simulink library "HDL_ieee_8021513"  (R2024a)
settings: Solver=FixedStepDiscrete  StartTime=0.0  StopTime=10.0  RelTol=1e-3
undefined symbols (not defined in the file or in its folder): Add, axiWidth, channelCyclicPrefixLen, channelDataCarriers, channelEstReference, channelLUT, channelOFDMSamples, channelScramblerInit, decimatorDelay, decimatorFilter, fPHY, frequencyOffsetTimeWindow, fs, headerBitsPerFec, headerBitsPerOFDMSymbol, headerBitsPerSubcarrier, headerCyclicPrefixLen, headerDataCarriers, headerOFDMSamples, headerScramblerInit, interpolatorDelay, interpolatorFilter, leftGuard, N, ncoCarrierFrequency, ncoWordLength, numDataCarriers, oversamplingFactor, payloadBitsPerFec, payloadScramblerInit, payloadWordsPerBlock0, peakDetectorThreshold, peakDetectorWindow, preambleCyclicPrefixLen, preambleDataCarriers, preambleLUT, preambleOFDMSamples, preambleScramblerInit, QAM, rightGuard, Shift
libraries: hdlsllib x198, $bdroot x80, whdlutilities x28, whdledac x10, whdlmod x7, simulink x4, dsphdlfiltering2 x2, dsphdlsigops2 x2, commhdlcrc x2, dspsigops x2, dspstat3 x2, commdigbbndam3 x2
(part 2 of 5)

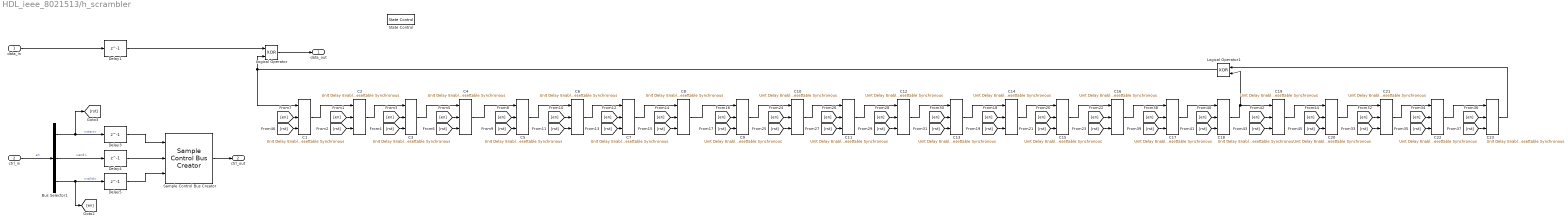
== system HDL_ieee_8021513/h_scrambler ==
  data_in : Inport
  ctrl_in : Inport  Port=2
  Bus Selector1 : BusSelector  OutputSignals=start,end,valid
  C{1,3,5,7,9,11,13,15,17,19,21,23} (12 alike) : hdlsllib/Discrete/Unit Delay Enabled Resettable Synchronous  InitialCondition=0  SampleTime=-1
  C{2,4,6,8,10,12,14,16,18,20,22} (11 alike) : hdlsllib/Discrete/Unit Delay Enabled Resettable Synchronous  InitialCondition=1  SampleTime=-1
  Delay{1,3..5} (4 alike) : Delay  DelayLength=1  InitialCondition=0  UseCircularBuffer=on
  Logical Operator : Logic  Operator=XOR  IconShape=distinctive  AllPortsSameDT=off  OutDataTypeStr=boolean
  Logical Operator1 : Logic  Operator=XOR  IconShape=distinctive  AllPortsSameDT=off  OutDataTypeStr=boolean
  Sample Control Bus Creator : whdlutilities/Sample Control Bus Creator
  State Control : StateControl  StateControl=Synchronous
  data_out : Outport
  ctrl_out : Outport  Port=2  VectorParamsAs1DForOutWhenUnconnected=off
  wires:
  Sample Control Bus Creator/1 -> ctrl_out/1
  Delay5/1 -> Sample Control Bus Creator/3
  Delay4/1 -> Sample Control Bus Creator/2
  Delay3/1 -> Sample Control Bus Creator/1
  Bus Selector1/3 -> Delay5/1, [en]  "<valid>"
  Bus Selector1/2 -> Delay4/1  "<end>"
  Bus Selector1/1 -> Delay3/1, [rst]  "<start>"
  C23/1 -> Logical Operator1/1
  [rst] -> C22/3
  C19/1 -> C20/1
  [en] -> C20/2
  [en] -> C21/2
  C21/1 -> C22/1
  [rst] -> C18/3
  [en] -> C17/2
  [rst] -> C19/3
  [rst] -> C21/3
  C17/1 -> C18/1
  C22/1 -> C23/1
  [en] -> C19/2
  [en] -> C18/2
  [en] -> C23/2
  [rst] -> C20/3
  [en] -> C22/2
  C16/1 -> C17/1
  [rst] -> C23/3
  [rst] -> C17/3
  C8/1 -> C9/1
  [rst] -> C15/3
  [en] -> C15/2
  [en] -> C14/2
  [rst] -> C16/3
  [en] -> C12/2
  [rst] -> C14/3
  C13/1 -> C14/1
  C11/1 -> C12/1
  [rst] -> C9/3
  [en] -> C10/2
  [en] -> C9/2
  C14/1 -> C15/1
  [en] -> C11/2
  [rst] -> C13/3
  C10/1 -> C11/1
  [rst] -> C10/3
  C12/1 -> C13/1
  [en] -> C13/2
  [rst] -> C11/3
  [en] -> C16/2
  [rst] -> C12/3
  C9/1 -> C10/1
  C15/1 -> C16/1
  [rst] -> C5/3
  [en] -> C6/2
  C6/1 -> C7/1
  [en] -> C8/2
  [rst] -> C6/3
  C5/1 -> C6/1
  [rst] -> C7/3
  C7/1 -> C8/1
  [rst] -> C8/3
  [en] -> C7/2
  [en] -> C5/2
  Delay1/1 -> Logical Operator/1
  data_in/1 -> Delay1/1
  ctrl_in/1 -> Bus Selector1/1  "en"
  Logical Operator/1 -> data_out/1
  [rst] -> C3/3
  [en] -> C3/2
  Logical Operator1/1 -> Logical Operator/2, C1/1
  [rst] -> C2/3
  C1/1 -> C2/1
  C3/1 -> C4/1
  [en] -> C1/2
  [rst] -> C1/3
  C4/1 -> C5/1
  [en] -> C4/2
  C2/1 -> C3/1
  [rst] -> C4/3
  [en] -> C2/2
  C20/1 -> C21/1
  C18/1 -> Logical Operator1/2, C19/1

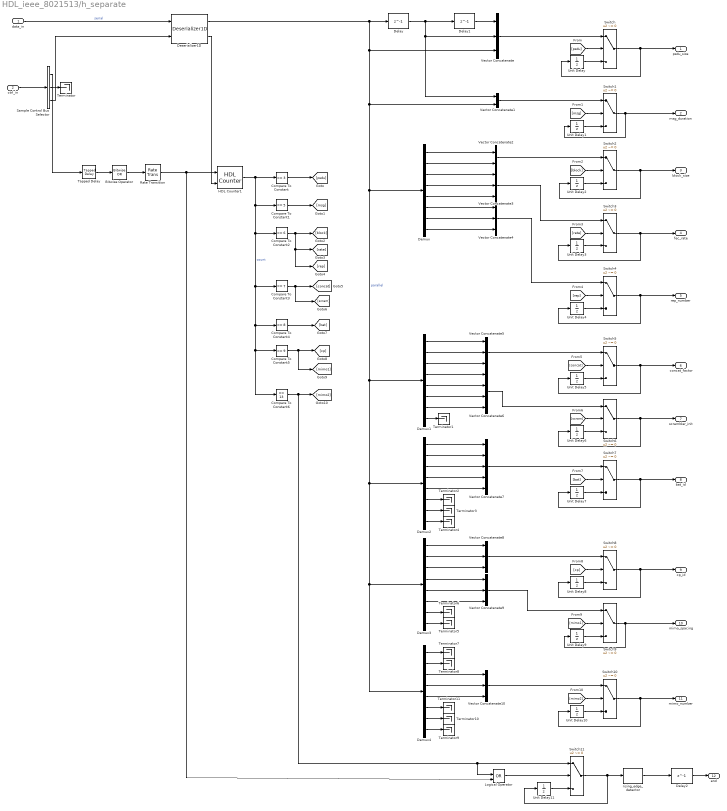
== system HDL_ieee_8021513/h_separate ==
  data_in : Inport
  ctrl_in : Inport  Port=2
  Bitwise Operator : simulink/Logic and Bit Operations/Bitwise Operator  logicop=OR  UseBitMask=off  BitMask=bin2dec('11011001')  BitMaskRealWorld=Stored Integer
      settings: LibrarySourceBlock=|
      | hdlsllib/Logic and Bit
      | Operations/Bitwise
      | Operator
  Compare To Constant : hdlsllib/Logic and Bit Operations/Compare To Constant  relop===  const=3  OutDataTypeStr=boolean
  Compare To Constant1 : hdlsllib/Logic and Bit Operations/Compare To Constant  relop===  const=5  OutDataTypeStr=boolean
  Compare To Constant2 : hdlsllib/Logic and Bit Operations/Compare To Constant  relop===  const=6  OutDataTypeStr=boolean
  Compare To Constant3 : hdlsllib/Logic and Bit Operations/Compare To Constant  relop===  const=7  OutDataTypeStr=boolean
  Compare To Constant4 : hdlsllib/Logic and Bit Operations/Compare To Constant  relop===  const=8  OutDataTypeStr=boolean
  Compare To Constant5 : hdlsllib/Logic and Bit Operations/Compare To Constant  relop===  const=9  OutDataTypeStr=boolean
  Compare To Constant6 : hdlsllib/Logic and Bit Operations/Compare To Constant  relop===  const=13  OutDataTypeStr=boolean
  Delay : Delay  DelayLength=1  InitialCondition=0  UseCircularBuffer=on
  Delay1 : Delay  DelayLength=1  InitialCondition=0  UseCircularBuffer=on
  Delay2 : Delay  DelayLength=1  InitialCondition=0  UseCircularBuffer=on
  Demux{,1..4} (5 alike) : Demux  Outputs=8
  Deserializer1D : hdlsllib/HDL Operations/Deserializer1D  Ratio=8  IdleCycles=0  InitialCondition=0  startIn=off  validIn=on  validOut=on  inputDataDimensions=-1  inputSampleTime=-1  inputSignalType=auto
  HDL Counter1 : hdlsllib/Sources/HDL Counter  CountType=Free running  CountInit=0  CountStep=1  CountMax=25  CountFromType=Initial value  CountFrom=0  CountResetPort=on  CountLoadPort=off  CountEnbPort=on  CountDirPort=off  CountHitOutputPort=off  CountDataType=Unsigned  CountWordLen=5  CountFracLen=0  CountSampTime=1
  Logical Operator : Logic  Operator=OR  IconShape=distinctive  AllPortsSameDT=off  OutDataTypeStr=boolean
  Rate Transition : RateTransition  OutPortSampleTimeOpt=Multiple of input port sample time  OutPortSampleTimeMultiple=8
  Sample Control Bus Selector : whdlutilities/Sample Control Bus Selector  OutputSignals=start,end,valid
  Switch{,1..11} (12 alike) : Switch  Criteria=u2 ~= 0  SaturateOnIntegerOverflow=off  InputSameDT=off
  Tapped Delay : simulink/Discrete/Tapped Delay  vinit=0.0  samptime=-1  NumDelays=8  DelayOrder=Oldest  includeCurrent=off
      settings: LibrarySourceBlock=hdlsllib/Discrete/Tapped Delay
  Terminator{,1..11} (12 alike) : Terminator
  Unit Delay{,1..11} (12 alike) : UnitDelay  SampleTime=-1  HasFrameUpgradeWarning=on
  Vector Concatenate{,3..5,8..10} (7 alike) : Concatenate  NumInputs=3
  Vector Concatenate1 : Concatenate
  Vector Concatenate2 : Concatenate
  Vector Concatenate6 : Concatenate  NumInputs=4
  Vector Concatenate7 : Concatenate  NumInputs=5
  rising_edge_detector : $bdroot/rising_edge_detector  SystemSampleTime=-1  VariantActivationTime=update diagram  AllowFlexibleInterface=on  Latency=0  AutoFrameSizeCalculation=off
  psdu_size : Outport
  msg_duration : Outport  Port=2
  block_size : Outport  Port=3
  fec_rate : Outport  Port=4
  rep_number : Outport  Port=5
  concat_factor : Outport  Port=6
  scrambler_init : Outport  Port=7
  bat_id : Outport  Port=8
  cp_id : Outport  Port=9
  mimo_spacing : Outport  Port=10
  mimo_number : Outport  Port=11
  end : Outport  Port=12  VectorParamsAs1DForOutWhenUnconnected=off
  wires:
  rising_edge_detector/1 -> Delay2/1
  Bitwise Operator/1 -> Rate Transition/1
  Tapped Delay/1 -> Bitwise Operator/1
  Delay2/1 -> end/1
  Logical Operator/1 -> Switch11/2
  Compare To Constant6/1 -> [mimo2], Switch11/1, Logical Operator/1
  Unit Delay11/1 -> Switch11/3
  Switch11/1 -> rising_edge_detector/1, Unit Delay11/1
  Vector Concatenate10/1 -> Switch10/1
  Demux4/5 -> Vector Concatenate10/3
  Demux4/4 -> Vector Concatenate10/2
  Demux4/3 -> Vector Concatenate10/1
  Demux4/6 -> Terminator11/1
  Demux4/7 -> Terminator10/1
  Demux4/8 -> Terminator9/1
  Demux4/2 -> Terminator8/1
  Demux4/1 -> Terminator7/1
  Vector Concatenate9/1 -> Switch9/1
  Vector Concatenate8/1 -> Switch8/1
  Demux3/3 -> Vector Concatenate8/3
  Demux3/2 -> Vector Concatenate8/2
  Demux3/1 -> Vector Concatenate8/1
  Demux3/6 -> Vector Concatenate9/3
  Demux3/5 -> Vector Concatenate9/2
  Demux3/4 -> Vector Concatenate9/1
  Demux3/7 -> Terminator6/1
  Demux3/8 -> Terminator5/1
  Vector Concatenate7/1 -> Switch7/1
  Demux2/5 -> Vector Concatenate7/5
  Demux2/4 -> Vector Concatenate7/4
  Demux2/3 -> Vector Concatenate7/3
  Demux2/2 -> Vector Concatenate7/2
  Demux2/1 -> Vector Concatenate7/1
  Demux2/8 -> Terminator4/1
  Demux2/7 -> Terminator3/1
  Demux2/6 -> Terminator2/1
  Vector Concatenate6/1 -> Switch6/1
  Demux1/8 -> Terminator1/1
  Demux1/7 -> Vector Concatenate6/4
  Demux1/6 -> Vector Concatenate6/3
  Demux1/5 -> Vector Concatenate6/2
  Demux1/4 -> Vector Concatenate6/1
  Vector Concatenate5/1 -> Switch5/1
  Demux1/3 -> Vector Concatenate5/3
  Demux1/2 -> Vector Concatenate5/2
  Demux1/1 -> Vector Concatenate5/1
  Vector Concatenate4/1 -> Switch4/1
  Demux/8 -> Vector Concatenate4/3
  Demux/7 -> Vector Concatenate4/2
  Demux/6 -> Vector Concatenate4/1
  Vector Concatenate3/1 -> Switch3/1
  Demux/5 -> Vector Concatenate3/3
  Demux/4 -> Vector Concatenate3/2
  Demux/3 -> Vector Concatenate3/1
  Vector Concatenate2/1 -> Switch2/1
  Demux/2 -> Vector Concatenate2/2
  Demux/1 -> Vector Concatenate2/1
  Sample Control Bus Selector/2 -> Terminator/1
  Vector Concatenate1/1 -> Switch1/1
  [mimo2] -> Switch10/2
  Switch10/1 -> Unit Delay10/1, mimo_number/1
  Unit Delay10/1 -> Switch10/3
  [mimo1] -> Switch9/2
  Switch9/1 -> Unit Delay9/1, mimo_spacing/1
  Unit Delay9/1 -> Switch9/3
  [cp] -> Switch8/2
  Switch8/1 -> Unit Delay8/1, cp_id/1
  Unit Delay8/1 -> Switch8/3
  [bat] -> Switch7/2
  Switch7/1 -> Unit Delay7/1, bat_id/1
  Unit Delay7/1 -> Switch7/3
  [scram] -> Switch6/2
  Switch6/1 -> Unit Delay6/1, scrambler_init/1
  Unit Delay6/1 -> Switch6/3
  [concat] -> Switch5/2
  Switch5/1 -> Unit Delay5/1, concat_factor/1
  Unit Delay5/1 -> Switch5/3
  [rep] -> Switch4/2
  Switch4/1 -> Unit Delay4/1, rep_number/1
  Unit Delay4/1 -> Switch4/3
  [rate] -> Switch3/2
  Switch3/1 -> Unit Delay3/1, fec_rate/1
  Unit Delay3/1 -> Switch3/3
  [block] -> Switch2/2
  Switch2/1 -> Unit Delay2/1, block_size/1
  Unit Delay2/1 -> Switch2/3
  Switch1/1 -> Unit Delay1/1, msg_duration/1
  Unit Delay1/1 -> Switch1/3
  [msg] -> Switch1/2
  [psdu] -> Switch/2
  Compare To Constant5/1 -> [cp], [mimo1]
  Compare To Constant4/1 -> [bat]
  Compare To Constant3/1 -> [concat], [scram]
  Compare To Constant2/1 -> [rep], [rate], [block]
  Compare To Constant1/1 -> [msg]
  Compare To Constant/1 -> [psdu]
  HDL Counter1/1 -> Compare To Constant/1, Compare To Constant1/1, Compare To Constant2/1, Compare To Constant3/1, Compare To Constant4/1, Compare To Constant5/1, Compare To Constant6/1  "count"
  Rate Transition/1 -> HDL Counter1/1, Logical Operator/2
  Deserializer1D/2 -> HDL Counter1/2
  Unit Delay/1 -> Switch/3
  Switch/1 -> psdu_size/1, Unit Delay/1
  Vector Concatenate/1 -> Switch/1
  Delay1/1 -> Vector Concatenate/1
  Delay/1 -> Delay1/1, Vector Concatenate/2, Vector Concatenate1/1
  Deserializer1D/1 -> Vector Concatenate/3, Vector Concatenate1/2, Demux/1, Demux1/1, Demux2/1, Demux3/1, Demux4/1, Delay/1  "parallel"
  data_in/1 -> Deserializer1D/1  "serial"
  Sample Control Bus Selector/1 -> Tapped Delay/1
  Sample Control Bus Selector/3 -> Deserializer1D/2
  ctrl_in/1 -> Sample Control Bus Selector/1

== system HDL_ieee_8021513/header_fec ==
  data_in : Inport
  ctrl_in : Inport  Port=2
  Hc_12H_B14 : whdledac/LDPC Encoder  ParityCheckMatrix=Hc_12H  BlockSize=14  SimulateUsing=Code generation
  data_out : Outport
  ctrl_out : Outport  Port=2
  next_frame : Outport  Port=3
  wires:
  ctrl_in/1 -> Hc_12H_B14/2
  data_in/1 -> Hc_12H_B14/1
  Hc_12H_B14/2 -> ctrl_out/1
  Hc_12H_B14/1 -> data_out/1
  Hc_12H_B14/3 -> next_frame/1

== system HDL_ieee_8021513/header_full ==
  new_frame : Inport
  psdu_size : Inport  Port=2
  msg_duration : Inport  Port=3
  block_size : Inport  Port=4
  fec_rate : Inport  Port=5
  rep_number : Inport  Port=6
  concat_factor : Inport  Port=7
  scrambler_init : Inport  Port=8
  bat_id : Inport  Port=9
  cp_id : Inport  Port=10
  mimo_spacing : Inport  Port=11
  mimo_number : Inport  Port=12
  h_crc : $bdroot/h_crc  SystemSampleTime=-1  VariantActivationTime=update diagram  AllowFlexibleInterface=on  Latency=0  AutoFrameSizeCalculation=off
  h_gen : $bdroot/h_gen  SystemSampleTime=-1  VariantActivationTime=update diagram  AllowFlexibleInterface=on  Latency=0  AutoFrameSizeCalculation=off
  h_repetition : $bdroot/h_repetition  SystemSampleTime=-1  VariantActivationTime=update diagram  AllowFlexibleInterface=on  Latency=0  AutoFrameSizeCalculation=off
  h_scrambler : $bdroot/h_scrambler  SystemSampleTime=-1  VariantActivationTime=update diagram  AllowFlexibleInterface=on  Latency=0  AutoFrameSizeCalculation=off
      settings: LibrarySourceBlock=|
      | hdlsllib/Ports &
      | Subsystems/Subsystem
  header_fec : $bdroot/header_fec  SystemSampleTime=-1  VariantActivationTime=update diagram  AllowFlexibleInterface=on  Latency=0  AutoFrameSizeCalculation=off
  header : Outport  VectorParamsAs1DForOutWhenUnconnected=off
  ctrl_out : Outport  Port=2  VectorParamsAs1DForOutWhenUnconnected=off
  next_frame : Outport  Port=3  VectorParamsAs1DForOutWhenUnconnected=off
  wires:
  h_scrambler/1 -> header_fec/1
  h_scrambler/2 -> header_fec/2
  header_fec/1 -> h_repetition/1  "dataOut"
  header_fec/2 -> h_repetition/2
  h_crc/2 -> h_scrambler/2
  h_crc/1 -> h_scrambler/1
  h_gen/2 -> h_crc/2
  h_gen/1 -> h_crc/1
  h_repetition/2 -> ctrl_out/1
  h_repetition/1 -> header/1
  new_frame/1 -> h_gen/1
  psdu_size/1 -> h_gen/2
  msg_duration/1 -> h_gen/3
  block_size/1 -> h_gen/4
  fec_rate/1 -> h_gen/5
  rep_number/1 -> h_gen/6
  concat_factor/1 -> h_gen/7
  scrambler_init/1 -> h_gen/8
  bat_id/1 -> h_gen/9
  cp_id/1 -> h_gen/10
  mimo_spacing/1 -> h_gen/11
  mimo_number/1 -> h_gen/12
  header_fec/3 -> next_frame/1

== system HDL_ieee_8021513/interpolator ==
  data_in : Inport
  valid_in : Inport  Port=2
  Delay : Delay  DelayLength=1  InitialCondition=0  UseCircularBuffer=on
  Delay1 : Delay  DelayLength=interpolatorDelay  InitialCondition=0  UseCircularBuffer=on
  Delay3 : Delay  DelayLength=(interpolatorDelay+1)/2  InitialCondition=0  UseCircularBuffer=on
  Delay4 : Delay  DelayLength=1  InitialCondition=0  UseCircularBuffer=on
  FIR Interpolator : dsphdlfiltering2/FIR Interpolator  Numerator=interpolatorFilter.Numerator  FilterStructure=Direct form systolic  InterpolationFactor=oversamplingFactor  NumCycles=oversamplingFactor  SimulateUsing=Code generation  roundingMode=Floor  overflowMode=off  CoefficientsDataTypeStr=fixdt(1,16,14)  OutputDataTypeStr=fixdt(1,16,14)  ResetInputPort=off  HDLGlobalReset=off
  Logical Operator : Logic  Operator=OR  IconShape=distinctive  AllPortsSameDT=off  OutDataTypeStr=boolean
  Logical Operator1 : Logic  IconShape=distinctive  AllPortsSameDT=off  OutDataTypeStr=boolean
  Logical Operator2 : Logic  IconShape=distinctive  AllPortsSameDT=off  OutDataTypeStr=boolean
  Logical Operator3 : Logic  Operator=NOT  IconShape=distinctive  AllPortsSameDT=off  OutDataTypeStr=boolean
  Terminator1 : Terminator
  Upsample : dspsigops/Upsample  FactorSource=Dialog parameter  N=oversamplingFactor  Nmax=16  phase=0  RateOptions=Allow multirate processing  ic=0  mode=Unused parameter value
      settings: LibrarySourceBlock=dsphdlsupportsigops/Upsample
  Upsample1 : dspsigops/Upsample  FactorSource=Dialog parameter  N=oversamplingFactor  Nmax=16  phase=0  RateOptions=Allow multirate processing  ic=0  mode=Unused parameter value
      settings: LibrarySourceBlock=dsphdlsupportsigops/Upsample
  falling_edge_detector : $bdroot/falling_edge_detector  SystemSampleTime=-1  VariantActivationTime=update diagram  AllowFlexibleInterface=on  Latency=0  AutoFrameSizeCalculation=off
  data_out : Outport  VectorParamsAs1DForOutWhenUnconnected=off
  valid_out : Outport  Port=2  VectorParamsAs1DForOutWhenUnconnected=off
  wires:
  data_in/1 -> Upsample/1
  FIR Interpolator/1 -> Delay4/1
  Upsample1/1 -> FIR Interpolator/2
  valid_in/1 -> Delay3/1, Logical Operator/1
  Logical Operator2/1 -> valid_out/1
  falling_edge_detector/1 -> Logical Operator3/1
  FIR Interpolator/3 -> Terminator1/1
  Delay1/1 -> Logical Operator1/2
  Delay3/1 -> Logical Operator/2
  Logical Operator/1 -> Upsample1/1
  Upsample/1 -> FIR Interpolator/1
  Logical Operator1/1 -> falling_edge_detector/1, Delay/1
  Delay4/1 -> data_out/1
  Logical Operator3/1 -> Logical Operator2/2
  FIR Interpolator/2 -> Delay1/1, Logical Operator1/1
  Delay/1 -> Logical Operator2/1

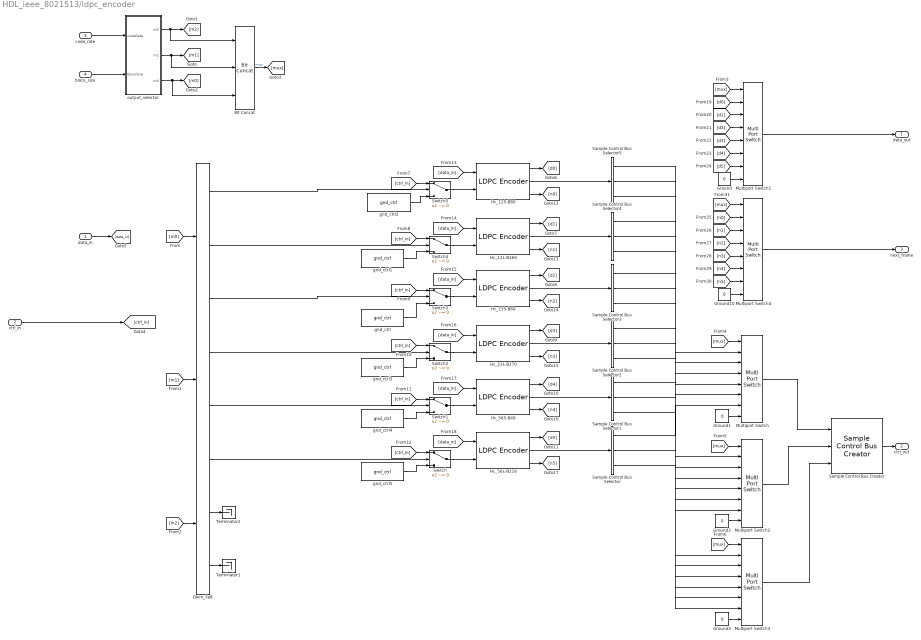
== system HDL_ieee_8021513/ldpc_encoder ==
  data_in : Inport
  ctrl_in : Inport  Port=2
  code_rate : Inport  Port=3
  block_size : Inport  Port=4
  Bit Concat : hdlsllib/Logic and Bit Operations/Bit Concat  numInputs=3
  Deco_3a8 : $bdroot/Deco_3a8  SystemSampleTime=-1  VariantActivationTime=update diagram  AllowFlexibleInterface=on  Latency=0  AutoFrameSizeCalculation=off
  Ground{,1..3,10} (5 alike) : Constant  Value=0  OutDataTypeStr=Inherit: Inherit via back propagation  SampleTime=-1
  Hc_12L-B360 : whdledac/LDPC Encoder  ParityCheckMatrix=Hc_12L  BlockSize=360  SimulateUsing=Code generation
  Hc_12S-B80 : whdledac/LDPC Encoder  ParityCheckMatrix=Hc_12S  BlockSize=80  SimulateUsing=Code generation
  Hc_23L-B270 : whdledac/LDPC Encoder  ParityCheckMatrix=Hc_23L  BlockSize=270  SimulateUsing=Code generation
  Hc_23S-B60 : whdledac/LDPC Encoder  ParityCheckMatrix=Hc_23S  BlockSize=60  SimulateUsing=Code generation
  Hc_56L-B216 : whdledac/LDPC Encoder  ParityCheckMatrix=Hc_56L  BlockSize=216  SimulateUsing=Code generation
  Hc_56S-B48 : whdledac/LDPC Encoder  ParityCheckMatrix=Hc_56S  BlockSize=48  SimulateUsing=Code generation
  Multiport Switch{,1..4} (5 alike) : MultiPortSwitch  DataPortOrder=Zero-based contiguous  Inputs=6  DataPortForDefault=Additional data port  DiagnosticForDefault=None  zeroidx=on  SaturateOnIntegerOverflow=off  InputSameDT=off
  Sample Control Bus Creator : whdlutilities/Sample Control Bus Creator
  Sample Control Bus Selector{,1..5} (6 alike) : whdlutilities/Sample Control Bus Selector  OutputSignals=start,end,valid
  Switch{,1..5} (6 alike) : Switch  Criteria=u2 ~= 0  SaturateOnIntegerOverflow=off  InputSameDT=off  OutDataTypeStr=Inherit: Same as first input
  Terminator1 : Terminator
  Terminator2 : Terminator
  gnd_ctrl{,1..5} (6 alike) : $bdroot/gnd_ctrl  SystemSampleTime=-1  VariantActivationTime=update diagram  AllowFlexibleInterface=on  Latency=0  AutoFrameSizeCalculation=off
  output_selector : Subsystem
  data_out : Outport
  ctrl_out : Outport  Port=2
  next_frame : Outport  Port=3
  wires:
  Multiport Switch1/1 -> data_out/1
  Switch/1 -> Hc_56L-B216/2
  Deco_3a8/8 -> Terminator1/1
  Deco_3a8/7 -> Terminator2/1
  Deco_3a8/6 -> Switch/2
  Switch5/1 -> Hc_12S-B80/2
  Switch4/1 -> Hc_12L-B360/2
  Switch3/1 -> Hc_23S-B60/2
  Switch2/1 -> Hc_23L-B270/2
  Switch1/1 -> Hc_56S-B48/2
  Deco_3a8/1 -> Switch5/2
  Deco_3a8/2 -> Switch4/2
  Deco_3a8/3 -> Switch3/2
  Deco_3a8/4 -> Switch2/2
  Deco_3a8/5 -> Switch1/2
  Hc_12L-B360/3 -> [n1]
  Hc_12S-B80/3 -> [n0]
  Hc_23S-B60/3 -> [n2]
  Hc_23L-B270/3 -> [n3]
  Hc_56S-B48/3 -> [n4]
  Hc_56L-B216/3 -> [n5]
  gnd_ctrl/1 -> Switch3/3
  Hc_56L-B216/2 -> Sample Control Bus Selector/1
  Sample Control Bus Selector/3 -> Multiport Switch3/7
  Sample Control Bus Selector/2 -> Multiport Switch2/7
  Sample Control Bus Selector/1 -> Multiport Switch/7
  Hc_56S-B48/2 -> Sample Control Bus Selector1/1
  Sample Control Bus Selector1/3 -> Multiport Switch3/6
  Sample Control Bus Selector1/2 -> Multiport Switch2/6
  Sample Control Bus Selector1/1 -> Multiport Switch/6
  Hc_23L-B270/2 -> Sample Control Bus Selector2/1
  Sample Control Bus Selector2/3 -> Multiport Switch3/5
  Sample Control Bus Selector2/2 -> Multiport Switch2/5
  Sample Control Bus Selector2/1 -> Multiport Switch/5
  Hc_23S-B60/2 -> Sample Control Bus Selector3/1
  Sample Control Bus Selector3/3 -> Multiport Switch3/4
  Sample Control Bus Selector3/2 -> Multiport Switch2/4
  Sample Control Bus Selector3/1 -> Multiport Switch/4
  Hc_12L-B360/2 -> Sample Control Bus Selector4/1
  Sample Control Bus Selector4/1 -> Multiport Switch/3
  Sample Control Bus Selector4/3 -> Multiport Switch3/3
  Sample Control Bus Selector4/2 -> Multiport Switch2/3
  Hc_12S-B80/2 -> Sample Control Bus Selector5/1
  Sample Control Bus Selector5/3 -> Multiport Switch3/2
  Sample Control Bus Selector5/2 -> Multiport Switch2/2
  Sample Control Bus Selector5/1 -> Multiport Switch/2
  Multiport Switch/1 -> Sample Control Bus Creator/1
  Multiport Switch2/1 -> Sample Control Bus Creator/2
  Multiport Switch3/1 -> Sample Control Bus Creator/3
  Sample Control Bus Creator/1 -> ctrl_out/1
  Ground/1 -> Multiport Switch1/8
  Ground1/1 -> Multiport Switch/8
  Ground2/1 -> Multiport Switch2/8
  Ground3/1 -> Multiport Switch3/8
  code_rate/1 -> output_selector/1(codeRate)
  block_size/1 -> output_selector/2(blockSize)
  output_selector/1(m2) -> Bit Concat/1, [m2]
  output_selector/3(m0) -> Bit Concat/3, [m0]
  output_selector/2(m1) -> Bit Concat/2, [m1]
  Bit Concat/1 -> [mux]  "mux"
  [m0] -> Deco_3a8/1
  [m1] -> Deco_3a8/2
  [m2] -> Deco_3a8/3
  [mux] -> Multiport Switch1/1
  [mux] -> Multiport Switch/1
  [mux] -> Multiport Switch2/1
  [mux] -> Multiport Switch3/1
  [ctrl_in] -> Switch5/1
  [ctrl_in] -> Switch4/1
  [ctrl_in] -> Switch3/1
  [ctrl_in] -> Switch2/1
  [ctrl_in] -> Switch1/1
  [ctrl_in] -> Switch/1
  data_in/1 -> [data_in]
  [data_in] -> Hc_12S-B80/1
  [data_in] -> Hc_12L-B360/1
  [data_in] -> Hc_23S-B60/1
  [data_in] -> Hc_23L-B270/1
  [data_in] -> Hc_56S-B48/1
  [data_in] -> Hc_56L-B216/1
  Hc_12S-B80/1 -> [d0]
  Hc_12L-B360/1 -> [d1]
  Hc_23S-B60/1 -> [d2]
  Hc_23L-B270/1 -> [d3]
  Hc_56S-B48/1 -> [d4]
  Hc_56L-B216/1 -> [d5]
  [d0] -> Multiport Switch1/2
  [d1] -> Multiport Switch1/3
  [d2] -> Multiport Switch1/4
  [d3] -> Multiport Switch1/5
  [d4] -> Multiport Switch1/6
  [d5] -> Multiport Switch1/7
  [n5] -> Multiport Switch4/7
  [n1] -> Multiport Switch4/3
  [n4] -> Multiport Switch4/6
  [n2] -> Multiport Switch4/4
  [mux] -> Multiport Switch4/1
  [n0] -> Multiport Switch4/2
  [n3] -> Multiport Switch4/5
  Multiport Switch4/1 -> next_frame/1
  Ground10/1 -> Multiport Switch4/8
  ctrl_in/1 -> [ctrl_in]
  gnd_ctrl1/1 -> Switch4/3
  gnd_ctrl2/1 -> Switch5/3
  gnd_ctrl3/1 -> Switch2/3
  gnd_ctrl4/1 -> Switch1/3
  gnd_ctrl5/1 -> Switch/3

== system HDL_ieee_8021513/next_frame_to_ready ==
  note: Given a next frame rising edge, this subsystem will generate a "ready" signal for the duration of "payloadWordsPerBlock0" clock cycles
  next_frame : Inport
  HDL Counter : hdlsllib/Sources/HDL Counter  CountType=Count limited  CountInit=0  CountStep=1  CountMax=payloadWordsPerBlock0-1  CountFromType=Initial value  CountFrom=0  CountResetPort=off  CountLoadPort=off  CountEnbPort=on  CountDirPort=off  CountHitOutputPort=on  CountDataType=Unsigned  CountWordLen=nextpow2(payloadWordsPerBlock0)  CountFracLen=0  CountSampTime=1
  Logical Operator2 : Logic  Operator=NOT  IconShape=distinctive  AllPortsSameDT=off  OutDataTypeStr=boolean
  Logical Operator3 : Logic  Operator=OR  IconShape=distinctive  AllPortsSameDT=off  OutDataTypeStr=boolean
  Terminator : Terminator
  Unit Delay Enabled Synchronous : hdlsllib/Discrete/Unit Delay Enabled Synchronous  InitialCondition=0.0  SampleTime=-1
  rising_edge_detector : $bdroot/rising_edge_detector  SystemSampleTime=-1  VariantActivationTime=update diagram  AllowFlexibleInterface=on  Latency=0  AutoFrameSizeCalculation=off
  ready : Outport  VectorParamsAs1DForOutWhenUnconnected=off
  wires:
  next_frame/1 -> rising_edge_detector/1
  HDL Counter/2 -> Logical Operator2/1, Logical Operator3/2
  Logical Operator3/1 -> Unit Delay Enabled Synchronous/2
  Unit Delay Enabled Synchronous/1 -> ready/1, HDL Counter/1
  HDL Counter/1 -> Terminator/1
  Logical Operator2/1 -> Unit Delay Enabled Synchronous/1
  rising_edge_detector/1 -> Logical Operator3/1

== system HDL_ieee_8021513/ofdm_demod ==
  data_in : Inport
  valid_in : Inport  Port=2
  cp_len : Inport  Port=3
  reset : Inport  Port=4
  Constant2 : Constant  Value=N  OutDataTypeStr=fixdt(0,9,0)  SampleTime=-1  LockScale=on
  Constant3 : Constant  Value=length(rightGuard)  OutDataTypeStr=fixdt(0,6,0)  SampleTime=-1  LockScale=on
  Constant4 : Constant  Value=length(leftGuard)  OutDataTypeStr=fixdt(0,6,0)  SampleTime=-1  LockScale=on
  OFDM Demodulator : whdlmod/OFDM Demodulator  OFDMParamsSource=Input port  MaxFFTLength=N  FFTLength=64  CPLength=16  NumLGsC=6  NumRGsC=5  CPFraction=off  CPFractionSource=Property  CPFractionValue=0.55  removeDCSubcarriers=off  enableResetInputPort=on  Normalize=off  RoundingMethod=Floor  SimulateUsing=Code generation
  data_out : Outport
  valid_out : Outport  Port=2
  ready : Outport  Port=3  VectorParamsAs1DForOutWhenUnconnected=off
  wires:
  reset/1 -> OFDM Demodulator/7
  Constant2/1 -> OFDM Demodulator/3
  Constant3/1 -> OFDM Demodulator/6
  Constant4/1 -> OFDM Demodulator/5
  data_in/1 -> OFDM Demodulator/1
  valid_in/1 -> OFDM Demodulator/2
  cp_len/1 -> OFDM Demodulator/4
  OFDM Demodulator/2 -> valid_out/1
  OFDM Demodulator/1 -> data_out/1
  OFDM Demodulator/3 -> ready/1

== system HDL_ieee_8021513/ofdm_modulator ==
  data_in : Inport
  valid_in : Inport  Port=2
  cp_len : Inport  Port=3
  Constant2 : Constant  Value=N  OutDataTypeStr=fixdt(0,9,0)  SampleTime=-1  LockScale=on
  Constant3 : Constant  Value=length(rightGuard)  OutDataTypeStr=fixdt(0,6,0)  SampleTime=-1  LockScale=on
  Constant4 : Constant  Value=length(leftGuard)  OutDataTypeStr=fixdt(0,6,0)  SampleTime=-1  LockScale=on
  OFDM Modulator : whdlmod/OFDM Modulator  OFDMParametersSource=Input Port  FFTLength=64  MaxFFTLength=N  CPLength=16  numLgSc=6  numRgSc=5  InsertDCNull=off  Windowing=off  WindowLength=4  MaxWindowLength=8  ResetInputPort=off  Normalize=on  RoundingMethod=Floor  SimulateUsing=Code generation
  data_out : Outport
  valid_out : Outport  Port=2
  ready : Outport  Port=3  VectorParamsAs1DForOutWhenUnconnected=off
  wires:
  Constant2/1 -> OFDM Modulator/3
  cp_len/1 -> OFDM Modulator/4
  Constant4/1 -> OFDM Modulator/5
  data_in/1 -> OFDM Modulator/1
  Constant3/1 -> OFDM Modulator/6
  OFDM Modulator/1 -> data_out/1
  OFDM Modulator/2 -> valid_out/1
  OFDM Modulator/3 -> ready/1
  valid_in/1 -> OFDM Modulator/2

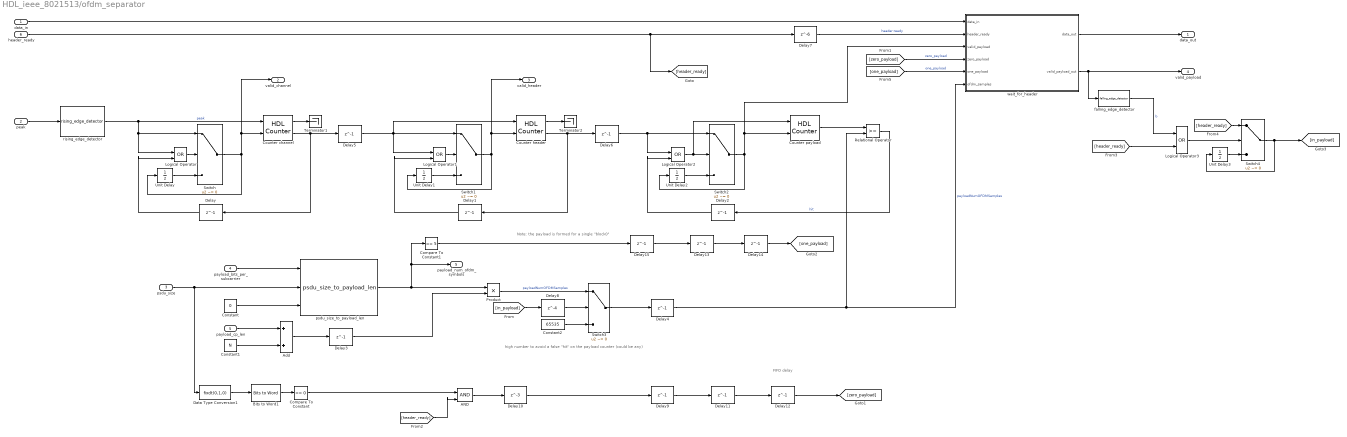
== system HDL_ieee_8021513/ofdm_separator ==
  note: FIFO delay
  note: Note: the payload is formed for a single "block0"
  note: high number to avoid a false "hit" on the payload counter (could be any)
  data_in : Inport
  peak : Inport  Port=2
  psdu_size : Inport  Port=3
  payload_bits_per_subcarrier : Inport  Port=4
  payload_cp_len : Inport  Port=5
  header_ready : Inport  Port=6
  AND : Logic  IconShape=distinctive  AllPortsSameDT=off  OutDataTypeStr=boolean
  Add : Sum  OutDataTypeStr=fixdt(0,16,0)
  Bits to Word1 : hdlsllib/Logic and Bit Operations/Bits to Word
  Compare To Constant : hdlsllib/Logic and Bit Operations/Compare To Constant  relop===  const=0  OutDataTypeStr=boolean
  Compare To Constant1 : hdlsllib/Logic and Bit Operations/Compare To Constant  relop===  const=5  OutDataTypeStr=boolean
  Constant : Constant  Value=0  OutDataTypeStr=boolean  SampleTime=-1
  Constant1 : Constant  Value=N  OutDataTypeStr=fixdt(0,9,0)  SampleTime=-1
  Constant2 : Constant  Value=65535  OutDataTypeStr=Inherit: Inherit via back propagation  SampleTime=-1
  Counter channel : hdlsllib/Sources/HDL Counter  CountType=Count limited  CountInit=0  CountStep=1  CountMax=channelOFDMSamples-2  CountFromType=Initial value  CountFrom=0  CountResetPort=on  CountLoadPort=off  CountEnbPort=on  CountDirPort=off  CountHitOutputPort=on  CountDataType=Unsigned  CountWordLen=nextpow2(channelOFDMSamples)  CountFracLen=0  CountSampTime=1
  Counter header : hdlsllib/Sources/HDL Counter  CountType=Count limited  CountInit=0  CountStep=1  CountMax=headerOFDMSamples-2  CountFromType=Initial value  CountFrom=0  CountResetPort=on  CountLoadPort=off  CountEnbPort=on  CountDirPort=off  CountHitOutputPort=on  CountDataType=Unsigned  CountWordLen=nextpow2(headerOFDMSamples)  CountFracLen=0  CountSampTime=1
  Counter payload : hdlsllib/Sources/HDL Counter  CountType=Free running  CountInit=2  CountStep=1  CountMax=headerOFDMSamples-1  CountFromType=Initial value  CountFrom=2  CountResetPort=on  CountLoadPort=off  CountEnbPort=on  CountDirPort=off  CountHitOutputPort=off  CountDataType=Unsigned  CountWordLen=32  CountFracLen=0  CountSampTime=1
  Data Type Conversion1 : DataTypeConversion  OutDataTypeStr=fixdt(0,1,0)  SaturateOnIntegerOverflow=off  RndMeth=Floor
  Delay{,1..6,9,11..15} (13 alike) : Delay  DelayLength=1  InitialCondition=0  UseCircularBuffer=on
  Delay10 : Delay  DelayLength=3  InitialCondition=0  UseCircularBuffer=on
  Delay7 : Delay  DelayLength=6  InitialCondition=0  UseCircularBuffer=on
  Delay8 : Delay  DelayLength=4  InitialCondition=0  UseCircularBuffer=on
  Logical Operator{,1..3} (4 alike) : Logic  Operator=OR  IconShape=distinctive  AllPortsSameDT=off  OutDataTypeStr=boolean
  Product : Product
  Relational Operator : RelationalOperator  OutDataTypeStr=boolean  InputSameDT=off
  Switch{,1..2,4} (4 alike) : Switch  Criteria=u2 ~= 0  SaturateOnIntegerOverflow=off  InputSameDT=off
  Switch3 : Switch  Criteria=u2 ~= 0  SaturateOnIntegerOverflow=off
  Terminator1 : Terminator
  Terminator2 : Terminator
  Unit Delay{,1..3} (4 alike) : UnitDelay  SampleTime=-1  HasFrameUpgradeWarning=on
  falling_edge_detector : $bdroot/falling_edge_detector  SystemSampleTime=-1  VariantActivationTime=update diagram  AllowFlexibleInterface=on  Latency=0  AutoFrameSizeCalculation=off
  psdu_size_to_payload_len : $bdroot/payload_full/psdu_size_to_payload_len  SystemSampleTime=-1  VariantActivationTime=update diagram  AllowFlexibleInterface=on  Latency=0  AutoFrameSizeCalculation=off
  rising_edge_detector : $bdroot/rising_edge_detector  SystemSampleTime=-1  VariantActivationTime=update diagram  AllowFlexibleInterface=on  Latency=0  AutoFrameSizeCalculation=off
  wait_for_header : Subsystem
  data_out : Outport  VectorParamsAs1DForOutWhenUnconnected=off
  valid_channel : Outport  Port=2
  valid_header : Outport  Port=3
  valid_payload : Outport  Port=4
  payload_num_ofdm_symbols : Outport  Port=5  VectorParamsAs1DForOutWhenUnconnected=off
  wires:
  peak/1 -> rising_edge_detector/1
  Counter channel/1 -> Terminator1/1
  Counter header/1 -> Terminator2/1
  Unit Delay/1 -> Switch/3
  Switch/1 -> valid_channel/1, Counter channel/2, Unit Delay/1
  Logical Operator/1 -> Switch/2
  Counter channel/2 -> Delay5/1, Delay/1
  Delay/1 -> Logical Operator/2
  Delay1/1 -> Logical Operator1/2
  Logical Operator1/1 -> Switch1/2
  Unit Delay1/1 -> Switch1/3
  Switch1/1 -> Unit Delay1/1, valid_header/1, Counter header/2
  Delay2/1 -> Logical Operator2/2
  Unit Delay2/1 -> Switch2/3
  Logical Operator2/1 -> Counter payload/1, Switch2/2
  Switch2/1 -> wait_for_header/3(valid_payload), Counter payload/2, Unit Delay2/1
  Counter header/2 -> Delay6/1, Delay1/1
  rising_edge_detector/1 -> Logical Operator/1, Switch/1, Counter channel/1  "peak"
  Constant1/1 -> Add/2
  payload_cp_len/1 -> Add/1
  Add/1 -> Delay3/1
  Relational Operator/1 -> Delay2/1  "hit"
  Counter payload/1 -> Relational Operator/1
  Delay5/1 -> Counter header/1, Logical Operator1/1, Switch1/1
  psdu_size/1 -> Data Type Conversion1/1, psdu_size_to_payload_len/2
  payload_bits_per_subcarrier/1 -> psdu_size_to_payload_len/1
  Constant/1 -> psdu_size_to_payload_len/3
  psdu_size_to_payload_len/1 -> Compare To Constant1/1, payload_num_ofdm_symbols/1, Product/1
  Delay3/1 -> Product/2
  data_in/1 -> wait_for_header/1(data_in)
  wait_for_header/1(data_out) -> data_out/1
  wait_for_header/2(valid_payload_out) -> valid_payload/1, falling_edge_detector/1
  Product/1 -> Switch3/1  "payloadNumOFDMSamples"
  Constant2/1 -> Switch3/3
  Switch3/1 -> Delay4/1
  Delay4/1 -> wait_for_header/6(ofdm_samples), Relational Operator/2  "payloadNumOFDMSamples"
  header_ready/1 -> [header_ready], Delay7/1
  Data Type Conversion1/1 -> Bits to Word1/1
  Bits to Word1/1 -> Compare To Constant/1
  [zero_payload] -> wait_for_header/4(zero_payload)  "zero_payload"
  [header_ready] -> AND/2
  AND/1 -> Delay10/1
  [in_payload] -> Delay8/1
  falling_edge_detector/1 -> Logical Operator3/1  "b"
  Delay6/1 -> Switch2/1, Logical Operator2/1
  Unit Delay3/1 -> Switch4/3
  Switch4/1 -> Unit Delay3/1, [in_payload]
  Logical Operator3/1 -> Switch4/2
  [header_ready] -> Logical Operator3/2
  [header_ready] -> Switch4/1
  Delay7/1 -> wait_for_header/2(header_ready)  "header:ready"
  Delay8/1 -> Switch3/2
  Delay9/1 -> Delay11/1
  [one_payload] -> wait_for_header/5(one_payload)  "one_payload"
  Compare To Constant/1 -> AND/1
  Delay11/1 -> Delay12/1
  Delay12/1 -> [zero_payload]
  Delay15/1 -> Delay13/1
  Compare To Constant1/1 -> Delay15/1
  Delay10/1 -> Delay9/1
  Delay13/1 -> Delay14/1
  Delay14/1 -> [one_payload]

== system HDL_ieee_8021513/ofdm_symbol_sync ==
  note: peakSync is synchronized with the first element of the channel
  note: Delay of find_peak = peakDetectorWindow
  data_in : Inport
  Delay : Delay  DelayLength=preambleOFDMSamples-100  InitialCondition=0  UseCircularBuffer=on
  Delay1 : Delay  DelayLength=128  InitialCondition=0  UseCircularBuffer=on
  Delay2 : Delay  DelayLength=100  InitialCondition=0  UseCircularBuffer=on
  find_peak : Subsystem
  frequency_offset_calculator : Subsystem
  m_cox : Subsystem
  data_out : Outport
  peak_sync : Outport  Port=2
  frequency_offset : Outport  Port=3  VectorParamsAs1DForOutWhenUnconnected=off
  M(d) : Outport  Port=4
  reset_ofdm : Outport  Port=5  VectorParamsAs1DForOutWhenUnconnected=off
  wires:
  Delay2/1 -> peak_sync/1
  data_in/1 -> m_cox/1(data_in)
  m_cox/2(M(d)) -> find_peak/2(M_in), M(d)/1
  m_cox/3(P(d)) -> Delay1/1
  m_cox/1(data_out) -> find_peak/1(data_in)
  find_peak/1(data_out) -> data_out/1
  find_peak/2(peak_sync) -> Delay/1, frequency_offset_calculator/1(peak_sync)
  Delay/1 -> Delay2/1, reset_ofdm/1
  Delay1/1 -> frequency_offset_calculator/2(P(d))
  frequency_offset_calculator/1(frequency_offset) -> frequency_offset/1

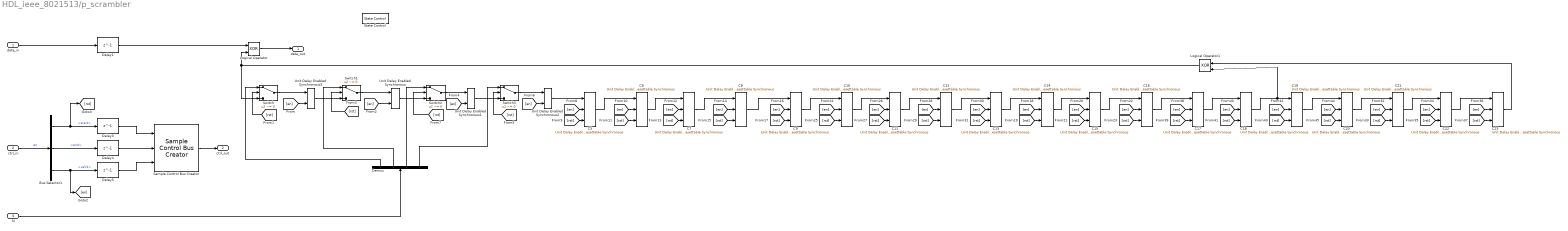
== system HDL_ieee_8021513/p_scrambler ==
  data_in : Inport
  ctrl_in : Inport  Port=2
  SI : Inport  Port=3
  Bus Selector1 : BusSelector  OutputSignals=start,end,valid
  C{5..23} (19 alike) : hdlsllib/Discrete/Unit Delay Enabled Resettable Synchronous  InitialCondition=1  SampleTime=-1
  Delay{1,3..5} (4 alike) : Delay  DelayLength=1  InitialCondition=0  UseCircularBuffer=on
  Demux : Demux
  Logical Operator : Logic  Operator=XOR  IconShape=distinctive  AllPortsSameDT=off  OutDataTypeStr=boolean
  Logical Operator1 : Logic  Operator=XOR  IconShape=distinctive  AllPortsSameDT=off  OutDataTypeStr=boolean
  Sample Control Bus Creator : whdlutilities/Sample Control Bus Creator
  State Control : StateControl  StateControl=Synchronous
  Switch{,1..3} (4 alike) : Switch  Criteria=u2 ~= 0  OutDataTypeStr=boolean  SaturateOnIntegerOverflow=off  InputSameDT=off
  Unit Delay Enabled Synchronous{,1..3} (4 alike) : hdlsllib/Discrete/Unit Delay Enabled Synchronous  InitialCondition=1  SampleTime=-1
  data_out : Outport
  ctrl_out : Outport  Port=2  VectorParamsAs1DForOutWhenUnconnected=off
  wires:
  Logical Operator1/1 -> Switch/3, Logical Operator/2
  Logical Operator/1 -> data_out/1
  ctrl_in/1 -> Bus Selector1/1  "en"
  data_in/1 -> Delay1/1
  Delay1/1 -> Logical Operator/1
  SI/1 -> Demux/1
  Demux/2 -> Switch1/1
  [en] -> Unit Delay Enabled Synchronous3/2
  [en] -> Unit Delay Enabled Synchronous/2
  [en] -> Unit Delay Enabled Synchronous1/2
  [en] -> Unit Delay Enabled Synchronous2/2
  [en] -> C5/2
  [en] -> C7/2
  [rst] -> C8/3
  C7/1 -> C8/1
  [rst] -> C7/3
  C5/1 -> C6/1
  [rst] -> C6/3
  [en] -> C8/2
  C6/1 -> C7/1
  [en] -> C6/2
  [rst] -> C5/3
  Unit Delay Enabled Synchronous2/1 -> C5/1
  C15/1 -> C16/1
  C9/1 -> C10/1
  [rst] -> C12/3
  [en] -> C16/2
  [rst] -> C11/3
  [en] -> C13/2
  C12/1 -> C13/1
  [rst] -> C10/3
  C10/1 -> C11/1
  [rst] -> C13/3
  [en] -> C11/2
  C14/1 -> C15/1
  [en] -> C9/2
  [en] -> C10/2
  [rst] -> C9/3
  C11/1 -> C12/1
  C13/1 -> C14/1
  [rst] -> C14/3
  [en] -> C12/2
  [rst] -> C16/3
  [en] -> C14/2
  [en] -> C15/2
  [rst] -> C15/3
  C8/1 -> C9/1
  [rst] -> C17/3
  [rst] -> C23/3
  C16/1 -> C17/1
  [en] -> C22/2
  C20/1 -> C21/1
  C18/1 -> Logical Operator1/2, C19/1
  [rst] -> C20/3
  [en] -> C23/2
  [en] -> C18/2
  [en] -> C19/2
  C22/1 -> C23/1
  C17/1 -> C18/1
  [rst] -> C21/3
  [rst] -> C19/3
  [en] -> C17/2
  [rst] -> C18/3
  C21/1 -> C22/1
  [en] -> C21/2
  [en] -> C20/2
  C19/1 -> C20/1
  [rst] -> C22/3
  C23/1 -> Logical Operator1/1
  [rst] -> Switch/2
  Demux/1 -> Switch/1
  Switch/1 -> Unit Delay Enabled Synchronous3/1
  Switch1/1 -> Unit Delay Enabled Synchronous/1
  [rst] -> Switch1/2
  Unit Delay Enabled Synchronous3/1 -> Switch1/3
  Switch2/1 -> Unit Delay Enabled Synchronous1/1
  Switch3/1 -> Unit Delay Enabled Synchronous2/1
  Unit Delay Enabled Synchronous1/1 -> Switch3/3
  [rst] -> Switch3/2
  Demux/4 -> Switch3/1
  Demux/3 -> Switch2/1
  Unit Delay Enabled Synchronous/1 -> Switch2/3
  [rst] -> Switch2/2
  Bus Selector1/1 -> [rst], Delay3/1  "<start>"
  Bus Selector1/2 -> Delay4/1  "<end>"
  Bus Selector1/3 -> [en], Delay5/1  "<valid>"
  Delay3/1 -> Sample Control Bus Creator/1
  Delay4/1 -> Sample Control Bus Creator/2
  Delay5/1 -> Sample Control Bus Creator/3
  Sample Control Bus Creator/1 -> ctrl_out/1

== system HDL_ieee_8021513/payload_full ==
  note: Note: careful when adding delays to signals "ready, valid or data" outside this block
  data_in : Inport
  valid_in : Inport  Port=2
  last_frame : Inport  Port=3
  new_frame : Inport  Port=4
  scrambler_init : Inport  Port=5
  fec_rate : Inport  Port=6
  block_size : Inport  Port=7
  bat_id : Inport  Port=8
  psdu_size : Inport  Port=9
  rep_number : Inport  Port=10
  Delay{,1..4} (5 alike) : Delay  DelayLength=1  InitialCondition=0  UseCircularBuffer=on
  Logical Operator : Logic  IconShape=distinctive  AllPortsSameDT=off  OutDataTypeStr=boolean
  Logical Operator1 : Logic  IconShape=distinctive  AllPortsSameDT=off  OutDataTypeStr=boolean
  Logical Operator5 : Logic  Operator=OR  IconShape=distinctive  AllPortsSameDT=off  OutDataTypeStr=boolean
  Rate Transition : RateTransition  OutPortSampleTimeOpt=Multiple of input port sample time  OutPortSampleTimeMultiple=axiWidth  OutPortSampleTime=1/fs
  Rate Transition{1..2,4,6} (4 alike) : RateTransition  OutPortSampleTimeOpt=Multiple of input port sample time  OutPortSampleTimeMultiple=1/axiWidth
  Rate Transition3 : RateTransition  OutPortSampleTimeOpt=Multiple of input port sample time  OutPortSampleTimeMultiple=1/axiWidth  OutPortSampleTime=1/axiWidth
  Rate Transition5 : RateTransition  OutPortSampleTimeOpt=Multiple of input port sample time  OutPortSampleTimeMultiple=1/axiWidth  OutPortSampleTime=1/axiWidth
  Serializer1D : hdlsllib/HDL Operations/Serializer1D  Ratio=axiWidth  IdleCycles=0  validIn=on  startOut=off  validOut=on  inputDataDimensions=-1  inputSampleTime=-1  inputSignalType=auto
  Switch1 : Switch  Criteria=u2 ~= 0  SaturateOnIntegerOverflow=off  InputSameDT=off
  Unit Delay1 : UnitDelay  SampleTime=-1  HasFrameUpgradeWarning=on
  Word to Bits : hdlsllib/Logic and Bit Operations/Word to Bits  maxWordLength=axiWidth
  batid_to_bits_per_subcarrier : $bdroot/batid_to_bits_per_subcarrier  SystemSampleTime=-1  VariantActivationTime=update diagram  AllowFlexibleInterface=on  Latency=0  AutoFrameSizeCalculation=off
  next_frame_to_ready : $bdroot/next_frame_to_ready  SystemSampleTime=-1  VariantActivationTime=update diagram  AllowFlexibleInterface=on  Latency=0  AutoFrameSizeCalculation=off
  p_scrambler : $bdroot/p_scrambler  SystemSampleTime=-1  VariantActivationTime=update diagram  AllowFlexibleInterface=on  Latency=0  AutoFrameSizeCalculation=off
      settings: LibrarySourceBlock=|
      | hdlsllib/Ports &
      | Subsystems/Subsystem
  payload_rep : $bdroot/payload_rep  SystemSampleTime=-1  VariantActivationTime=update diagram  AllowFlexibleInterface=on  Latency=0  AutoFrameSizeCalculation=off
  psdu_size_to_payload_len : Subsystem
  puncturer : $bdroot/puncturer  SystemSampleTime=-1  VariantActivationTime=update diagram  AllowFlexibleInterface=on  Latency=0  AutoFrameSizeCalculation=off
  reduced_ldpc : $bdroot/reduced_ldpc  SystemSampleTime=-1  VariantActivationTime=update diagram  AllowFlexibleInterface=on  Latency=0  AutoFrameSizeCalculation=off
  tone_mapping : $bdroot/tone_mapping  SystemSampleTime=-1  VariantActivationTime=update diagram  AllowFlexibleInterface=on  Latency=0  AutoFrameSizeCalculation=off
  valid_to_ctrl : $bdroot/valid_to_ctrl  SystemSampleTime=-1  VariantActivationTime=update diagram  AllowFlexibleInterface=on  Latency=0  AutoFrameSizeCalculation=off
  payload : Outport  VectorParamsAs1DForOutWhenUnconnected=off
  ctrl_out : Outport  Port=2  VectorParamsAs1DForOutWhenUnconnected=off
  ready : Outport  Port=3  VectorParamsAs1DForOutWhenUnconnected=off
  len_in_ofdm_symbols : Outport  Port=4  VectorParamsAs1DForOutWhenUnconnected=off
  bits_per_subcarrier : Outport  Port=5  VectorParamsAs1DForOutWhenUnconnected=off
  wires:
  block_size/1 -> Rate Transition3/1
  fec_rate/1 -> Rate Transition2/1
  p_scrambler/2 -> reduced_ldpc/2
  reduced_ldpc/2 -> puncturer/2
  p_scrambler/1 -> reduced_ldpc/1
  puncturer/2 -> payload_rep/2
  puncturer/1 -> payload_rep/1
  scrambler_init/1 -> Rate Transition1/1
  reduced_ldpc/1 -> puncturer/1  "dataOut"
  Delay/1 -> p_scrambler/1
  valid_to_ctrl/1 -> p_scrambler/2
  Serializer1D/2 -> valid_to_ctrl/1
  Serializer1D/1 -> Delay/1
  Word to Bits/1 -> Serializer1D/1
  Delay1/1 -> Rate Transition/1
  reduced_ldpc/3 -> Delay1/1
  next_frame_to_ready/1 -> Delay2/1, ready/1  "ready"
  Logical Operator/1 -> Serializer1D/2
  data_in/1 -> Delay4/1
  valid_in/1 -> Delay3/1
  Rate Transition/1 -> Logical Operator1/2
  Logical Operator1/1 -> next_frame_to_ready/1
  Unit Delay1/1 -> Switch1/3
  Switch1/1 -> Logical Operator1/1, Unit Delay1/1
  Logical Operator5/1 -> Switch1/2
  new_frame/1 -> Rate Transition6/1, Switch1/1, Logical Operator5/1
  last_frame/1 -> Logical Operator5/2
  Delay2/1 -> Logical Operator/1
  Delay4/1 -> Word to Bits/1
  Delay3/1 -> Logical Operator/2
  Rate Transition1/1 -> p_scrambler/3
  Rate Transition2/1 -> reduced_ldpc/3
  Rate Transition3/1 -> reduced_ldpc/4
  tone_mapping/2 -> ctrl_out/1
  payload_rep/2 -> tone_mapping/2  "ctrl_in"
  payload_rep/1 -> tone_mapping/1
  tone_mapping/1 -> payload/1
  batid_to_bits_per_subcarrier/1 -> psdu_size_to_payload_len/1(bits_per_subcarrier), Rate Transition4/1
  bat_id/1 -> batid_to_bits_per_subcarrier/1
  psdu_size/1 -> psdu_size_to_payload_len/2(psdu_size)
  rep_number/1 -> psdu_size_to_payload_len/3(rep_number)
  psdu_size_to_payload_len/1(payload_len_in_ofdm_symbols) -> Rate Transition5/1
  Rate Transition4/1 -> bits_per_subcarrier/1, tone_mapping/3  "bits_per_subcarrier"
  Rate Transition5/1 -> len_in_ofdm_symbols/1, tone_mapping/4  "len_in_ofdm_symbols"
  Rate Transition6/1 -> [new_frame]
  [new_frame] -> tone_mapping/5

== system HDL_ieee_8021513/payload_rep ==
  data_in : Inport
  ctrl_in : Inport  Port=2
  data_out : Outport
  ctrl_out : Outport  Port=2
  wires:
  data_in/1 -> data_out/1
  ctrl_in/1 -> ctrl_out/1

== system HDL_ieee_8021513/peak_detector ==
  note: TODO: local peak not working correctly
  note: This block has a latency of 19 clock cycles
  dataIn : Inport
  local_peak : Subsystem
  s1_index : Subsystem
  peak_sync : Outport
  wires:
  s1_index/1(indexes) -> local_peak/1(index)
  s1_index/2(Output) -> local_peak/2(dataIn)
  dataIn/1 -> s1_index/1(dataIn)
  local_peak/1(peak_sync) -> peak_sync/1

== system HDL_ieee_8021513/preamble_gen ==
  new_frame : Inport
  Delay : Delay  DelayLength=1  InitialCondition=0  UseCircularBuffer=on
  Direct Lookup Table (n-D) : LookupNDDirect  NumberOfTableDimensions=1  Table=preambleLUT  DiagnosticForOutOfRangeInput=Error  RemoveProtectionInput=on  TableDataTypeStr=boolean
  HDL Counter : hdlsllib/Sources/HDL Counter  CountType=Count limited  CountInit=0  CountStep=1  CountMax=length(preambleLUT)-1  CountFromType=Initial value  CountFrom=0  CountResetPort=off  CountLoadPort=off  CountEnbPort=on  CountDirPort=off  CountHitOutputPort=on  CountDataType=Unsigned  CountWordLen=12  CountFracLen=0  CountSampTime=1
  Logical Operator : Logic  Operator=NOT  IconShape=distinctive  AllPortsSameDT=off  OutDataTypeStr=boolean
  Logical Operator1 : Logic  Operator=OR  IconShape=distinctive  AllPortsSameDT=off  OutDataTypeStr=boolean
  Unit Delay Enabled Synchronous : hdlsllib/Discrete/Unit Delay Enabled Synchronous  InitialCondition=0.0  SampleTime=-1
  valid_to_ctrl : $bdroot/valid_to_ctrl  SystemSampleTime=-1  VariantActivationTime=update diagram  AllowFlexibleInterface=on  Latency=0  AutoFrameSizeCalculation=off
  data_out : Outport
  ctrl_out : Outport  Port=2
  wires:
  HDL Counter/1 -> Direct Lookup Table (n-D)/1
  Logical Operator/1 -> Unit Delay Enabled Synchronous/1
  HDL Counter/2 -> Logical Operator/1, Logical Operator1/2
  Logical Operator1/1 -> Unit Delay Enabled Synchronous/2
  new_frame/1 -> Logical Operator1/1
  Direct Lookup Table (n-D)/1 -> Delay/1
  Unit Delay Enabled Synchronous/1 -> valid_to_ctrl/1, HDL Counter/1
  valid_to_ctrl/1 -> ctrl_out/1
  Delay/1 -> data_out/1

== system HDL_ieee_8021513/puncturer ==
  data_in : Inport
  ctrl_in : Inport  Port=2
  data_out : Outport
  ctrl_out : Outport  Port=2
  wires:
  data_in/1 -> data_out/1
  ctrl_in/1 -> ctrl_out/1

== system HDL_ieee_8021513/qam_demod ==
  note: Note: using not a defailt QAM constellation results in an error while doing the HDL Code Generation
  data_in : Inport
  valid_in : Inport  Port=2
  bits_per_subcarrier : Inport  Port=3
  Constant{1..2,4..5} (4 alike) : Constant  Value=[0; 0; 0; 0]  VectorParams1D=off  OutDataTypeStr=Inherit: Inherit via back propagation  SampleTime=-1  LockScale=on
  Delay : Delay  DelayLength=1  InitialCondition=0  UseCircularBuffer=on
  Delay1 : Delay  DelayLength=1  InitialCondition=0  UseCircularBuffer=on
  Delay2 : Delay  DelayLength=0  InitialCondition=0  UseCircularBuffer=on
  Delay3 : Delay  DelayLength=1  InitialCondition=0  UseCircularBuffer=on
  Delay4 : Delay  DelayLength=0  InitialCondition=0  UseCircularBuffer=on
  Delay5 : Delay  DelayLength=6  InitialCondition=0  UseCircularBuffer=on
  Delay7 : Delay  DelayLength=6  InitialCondition=0  UseCircularBuffer=on
  Multiport Switch : MultiPortSwitch  DataPortOrder=Zero-based contiguous  Inputs=8  zeroidx=on  OutDataTypeStr=Inherit: Same as first data input  SaturateOnIntegerOverflow=off
  Symbol Demodulator : whdlmod/Symbol Demodulator  ModulationSource=Property  ModulationScheme=BPSK  MaxModulation=256-QAM  ConstOrder=Default  ConstMap=[ 2, 3, 1, 0, 6, 7, 5, 4, 14, 15, 13, 12, 10, 11, 9, 8 ]  DecisionType=Approximate log-likelihood ratio  PhaseOffset=0  OutputType=Vector  NormMethod=Unit average power  MinSymDistance=2  NoiseVariance=off  SimulateUsing=Code generation
  Symbol Demodulator1 : whdlmod/Symbol Demodulator  ModulationSource=Property  ModulationScheme=QPSK  MaxModulation=256-QAM  ConstOrder=Default  ConstMap=[ 2, 3, 1, 0, 6, 7, 5, 4, 14, 15, 13, 12, 10, 11, 9, 8 ]  DecisionType=Approximate log-likelihood ratio  PhaseOffset=-pi/4  OutputType=Vector  NormMethod=Unit average power  MinSymDistance=2  NoiseVariance=off  SimulateUsing=Code generation
  Symbol Demodulator2 : whdlmod/Symbol Demodulator  ModulationSource=Property  ModulationScheme=16-QAM  MaxModulation=256-QAM  ConstOrder=Default  ConstMap=qamFourBits.'  DecisionType=Approximate log-likelihood ratio  PhaseOffset=pi/2  OutputType=Vector  NormMethod=Unit average power  MinSymDistance=2  NoiseVariance=off  SimulateUsing=Code generation
  Terminator : Terminator
  Terminator1 : Terminator
  Terminator2 : Terminator
  to_12bit_integer : Subsystem
  data_out : Outport
  valid_out : Outport  Port=2  VectorParamsAs1DForOutWhenUnconnected=off
  wires:
  Delay/1 -> data_out/1
  to_12bit_integer/1(1bit_out) -> Multiport Switch/3, Multiport Switch/2
  Constant1/1 -> Multiport Switch/7
  bits_per_subcarrier/1 -> Delay7/1
  Delay1/1 -> valid_out/1
  Constant2/1 -> Multiport Switch/5
  Constant5/1 -> Multiport Switch/9
  valid_in/1 -> Delay5/1, Symbol Demodulator/2, Symbol Demodulator1/2, Symbol Demodulator2/2
  Multiport Switch/1 -> Delay/1
  Delay7/1 -> Multiport Switch/1
  Constant4/1 -> Multiport Switch/8
  data_in/1 -> Symbol Demodulator2/1, Symbol Demodulator1/1, Symbol Demodulator/1
  Symbol Demodulator/1 -> Delay2/1
  Symbol Demodulator1/1 -> Delay3/1
  Symbol Demodulator2/1 -> Delay4/1
  Symbol Demodulator2/2 -> Terminator/1
  Symbol Demodulator/2 -> Terminator1/1
  Symbol Demodulator1/2 -> Terminator2/1
  Delay5/1 -> Delay1/1
  Delay2/1 -> to_12bit_integer/1(1bit)
  Delay3/1 -> to_12bit_integer/2(2bit)
  Delay4/1 -> to_12bit_integer/3(4bit)
  to_12bit_integer/3(4bit_out) -> Multiport Switch/6
  to_12bit_integer/2(2bit_out) -> Multiport Switch/4
